simulink model "ADC_Capture_4x4_IQ_DDR4"  (R2019b)
settings: Solver=FixedStepDiscrete  StartTime=0.0  StopTime=inf  RelTol=1e-3
InitFcn:
  | init_ADC_Capture_4x4_IQ_DDR4
values from neighbouring files (symbols this model uses):
  Fs = ConverterSamplingRate/DDC_DUC_factor    (= 512000000)    [init_ADC_Capture_4x4_IQ_DDR4.m]
  N = 14    [init_ADC_Capture_4x4_IQ_DDR4.m]
  sim_CaptureLength = CaptureLength    (= 4096)    [init_ADC_Capture_4x4_IQ_DDR4.m]
  sim_RdFrameSize = 64    [init_ADC_Capture_4x4_IQ_DDR4.m]
  sim_RdNumFrames = ceil(sim_CaptureLength/sim_RdFrameSize)    [init_ADC_Capture_4x4_IQ_DDR4.m]
undefined symbols (not defined in the file or in its folder): config, DDR, Fo
libraries: hdlsllib x35, simulink x20, ddr4_behavioral_mdl x1, AXIDMALib x1, dsphdlsigops x1
(part 3 of 3)

== matlab function ADC_Capture_4x4_IQ_DDR4/DDR4 Model/DDR3/rdLogic/rd_control ==
  data: axi_rd_add input; axi_rd_len input; axi_rd_val input; axi_rd_ready input; ram_rd_addr output; ram_rd_val output boolean; toggle parameter; WR_RD_DATAWIDTH parameter
function [ram_rd_addr, ram_rd_val] = rd_add_gen(axi_rd_add,axi_rd_len, axi_rd_val,axi_rd_ready,toggle, WR_RD_DATAWIDTH)

%%%%%%%%%%%%%%%%%%%%%%%%%%%%%%%%%%%%%%%%%%%%%%%%%%%%%%
%%%Reg declaration
%RAM address generation counter
persistent ram_rd_cnt;

RD_BYTE_STRIDE = uint32(WR_RD_DATAWIDTH/8);

if(isempty(ram_rd_cnt))
    ram_rd_cnt = fi(0,0,32,0);%uint32(0);
end

%read response ack
persistent reg_rd_ack;

if(isempty(reg_rd_ack))
    reg_rd_ack = false;
end

%read status
persistent rd_progress;

if(isempty(rd_progress))
    rd_progress = false;
end

%read addr valid flag 
persistent rd_addr_val;

if(isempty(rd_addr_val))
    rd_addr_val = false;
end

%read addr valid flag 
persistent rd_addr_val_toggle;

if(isempty(rd_addr_val_toggle))
    rd_addr_val_toggle = false;
end

%start address and length of read burst latch
persistent start_addr;
if(isempty(start_addr))
    start_addr = fi(0,0,32,0);
end

persistent leng_latch;
if(isempty(leng_latch))
    leng_latch = fi(1,0,32,0);
end

%%%%%%%%%%%%%%%%%%%%%%%%%%%%%%%%%%%%%%%%%%%%%%%
%output
ram_rd_addr = (ram_rd_cnt);
ram_rd_val = (rd_addr_val);
%%%%%%%%%%%%%%%%%%%%%%%%%%%%%%%%%%%%%%%%%%%%%%%
if((reg_rd_ack == true)&&(axi_rd_ready == true))
    ram_rd_cnt = fi(start_addr,0,32,0);%uint32(start_addr );
    rd_addr_val = true;
elseif((rd_progress == true)&&(axi_rd_ready == true))
    
    if(rd_addr_val_toggle == true)
       ram_rd_cnt = fi(ram_rd_cnt + 1,0,32,0);%uint32(ram_rd_cnt + 1);
       rd_addr_val = true;
    else
       rd_addr_val = false;
   
    end
    if(toggle)
       rd_addr_val_toggle = ~(rd_addr_val_toggle);
    else
       rd_addr_val_toggle = true;
    end
elseif((rd_progress == false))  
    ram_rd_cnt = fi(0,0,32,0);%uint32(0) ;
    rd_addr_val = false;
else
    rd_addr_val = false;
end


%read progress flag
if((reg_rd_ack)&&(fi(ram_rd_cnt-start_addr,0,32,0)<fi(leng_latch-1,0,32,0)))
    rd_progress = true;
elseif(fi(ram_rd_cnt-start_addr,0,32,0)==fi(leng_latch-1,0,32,0))
    rd_progress = false;
end


%start address , length of burst latching
if(axi_rd_val)
    leng_latch(:) = axi_rd_len;
    start_addr(:) = axi_rd_add/RD_BYTE_STRIDE;
    reg_rd_ack = true;
else
    reg_rd_ack = false;
end

== matlab function ADC_Capture_4x4_IQ_DDR4/DDR4 Model/DDR3/wrLogic/Wr_control/MATLAB Function ==
  data: axi_wr_en input; wr_leng output; axi_wr_length input; wr_ack input
function wr_leng = addr_latch(axi_wr_en,axi_wr_length,wr_ack)
%#codegen

persistent axi_wr_en_d1;
if(isempty(axi_wr_en_d1))
axi_wr_en_d1 = false;
end

persistent reg_len;
if(isempty(reg_len))
    reg_len = fi(0,0,32,0);%uint32(0);
end


persistent reg_len_d1;
if(isempty(reg_len_d1))
    reg_len_d1 = fi(0,0,32,0);%uint32(0);
end

reg_len_d1 = reg_len;
wr_leng = reg_len;

if((axi_wr_en==true)&&(axi_wr_en_d1==false)&&(reg_len_d1==0)) 
  reg_len= fi(axi_wr_length,0,32,0);%axi_wr_length;
elseif(wr_ack)
  reg_len= fi(0,0,32,0);%uint32(0);    
end

axi_wr_en_d1 = axi_wr_en;

== matlab function ADC_Capture_4x4_IQ_DDR4/HDL_IP/DDR_Capture_Logic/DDR Write Conroller ==
  data: ram_addr output; ddr_write_done output; burst_len input; start input boolean; data_avail input; wr_ready input; wr_addr output; wr_len output; wr_valid output; wr_complete input; wasted_cycle_cnt output
function [ram_addr, ddr_write_done, wr_addr, wr_len, wr_valid,wasted_cycle_cnt] = ...
    fcn(burst_len, start, data_avail, wr_ready, wr_complete)

[ram_addr, ddr_write_done, wr_addr, wr_len, wr_valid, wasted_cycle_cnt] = ...
    controller.hdlcoder_external_memory_write_ctrl_custom(burst_len, start, data_avail, wr_ready, wr_complete);

end

== matlab function ADC_Capture_4x4_IQ_DDR4/HDL_IP/DDR_Capture_Logic/DataCaptureFIFO/FIFOWriteControl/MATLAB Function ==
  data: count_out output; DDRCaptureFIFOPush output; ADC_Valid input; RxStart input; CaptureLength input; FIFO_Full input; DDRCaptureFIFOActive output; FIFODropCount output
function [count_out, DDRCaptureFIFOPush, DDRCaptureFIFOActive, FIFODropCount] = capture_fifo_ctrl(ADC_Valid, RxStart, CaptureLength, FIFO_Full)

[count_out, DDRCaptureFIFOPush, DDRCaptureFIFOActive, FIFODropCount] = ...
    controller.capture_fifo(ADC_Valid, RxStart, CaptureLength, FIFO_Full)

end

== matlab function ADC_Capture_4x4_IQ_DDR4/HDL_IP/DDR_Capture_Logic/DDR Read Conroller ==
  data: valid_out output; count_out output; ddr_read_done output; burst_len input; rd_addr_in input; start input boolean; rd_aready input; rd_dvalid input; rd_addr output; rd_len output; rd_avalid output; ToggleTLAST output; debug_state output
function [valid_out,...
          count_out,...
          ddr_read_done,...
          rd_addr,...
          rd_len,...
          rd_avalid,...
          ToggleTLAST,...
          debug_state] = AXI4M_Rd(burst_len, rd_addr_in, start, rd_aready, rd_dvalid)

[valid_out, count_out, ddr_read_done, rd_addr, rd_len, rd_avalid,...
  ToggleTLAST, debug_state] = ...
  controller.pl_ddr_read_ctrl_original(burst_len, rd_addr_in, start, rd_aready, rd_dvalid)



end

== matlab function ADC_Capture_4x4_IQ_DDR4/read_ctrl Function ==
  data: wr_count input; rd_len output; rd_count input; rd_addr output; rd_trigger output; sim_CaptureLength parameter; sim_RdFrameSize parameter; DDRDataWidth input
function [rd_len, rd_addr, rd_trigger] = ...
    read_ctrl(wr_count, rd_count, sim_CaptureLength, sim_RdFrameSize, DDRDataWidth)

DATA_WIDTH_BYTES = DDRDataWidth/8;
WR_FRAME_SIZE = sim_CaptureLength;
RD_FRAME_SIZE = sim_RdFrameSize;

NUM_RD_FRAMES = ceil(WR_FRAME_SIZE/RD_FRAME_SIZE);
RD_ADDR_INC = RD_FRAME_SIZE*DATA_WIDTH_BYTES;

STATE_IDLE = 0;
STATE_READ_INIT = 1;
STATE_READ_WAIT = 2;

persistent wr_count_last rd_count_last next_state frame_count addr
if isempty(wr_count_last)
    wr_count_last = uint32(0);
    rd_count_last = uint32(0);
    frame_count = 0;
    addr = uint32(0);
    next_state = STATE_IDLE;
end

state = next_state;

rd_len = uint32(RD_FRAME_SIZE);
rd_addr = uint32(addr);
rd_trigger = (state == STATE_READ_INIT);

switch state
    
    case STATE_IDLE
        if wr_count > wr_count_last
            wr_count_last(:) = wr_count;
            next_state = STATE_READ_INIT;
            frame_count = 0;
            addr = uint32(0);
        end
        
    case STATE_READ_INIT
        next_state = STATE_READ_WAIT;
        
    case STATE_READ_WAIT
        if rd_count > rd_count_last
            
            rd_count_last(:) = rd_count;
            
            frame_count = frame_count + 1;
            
            if frame_count == NUM_RD_FRAMES
                next_state = STATE_IDLE;
            else
                next_state = STATE_READ_INIT;
                addr = addr + uint32(RD_ADDR_INC);
            end
            
        end
        
    otherwise
        next_state = STATE_IDLE;
end

== matlab function ADC_Capture_4x4_IQ_DDR4/HDL_IP/NCO_Transmit1/ScaleIQ and bit concat/HDL Flip1 ==
  data: u input; y output
function y = hdlflip(u)

N  = coder.const(numel(u));

out = zeros(size(u),'like',u);

coder.unroll();
for ii=1:N
    out(ii) = u(N-ii+1);
end
    
y = out;

== matlab function ADC_Capture_4x4_IQ_DDR4/HDL_IP/NCO_Transmit1/ScaleIQ and bit concat/HDL Flip2 ==
  data: u input; y output
function y = hdlflip(u)

N  = coder.const(numel(u));

out = zeros(size(u),'like',u);

coder.unroll();
for ii=1:N
    out(ii) = u(N-ii+1);
end
    
y = out;
